simulink model "matlab_simulation"  (R2015b)
settings: Solver=VariableStepAuto  StartTime=0  StopTime=0.8  FixedStep=0.001  RelTol=1e-3
libraries: fl_lib x14, nesl_utility x8, elec_lib x5
settings Model: Creator=User  LastModifiedBy=User

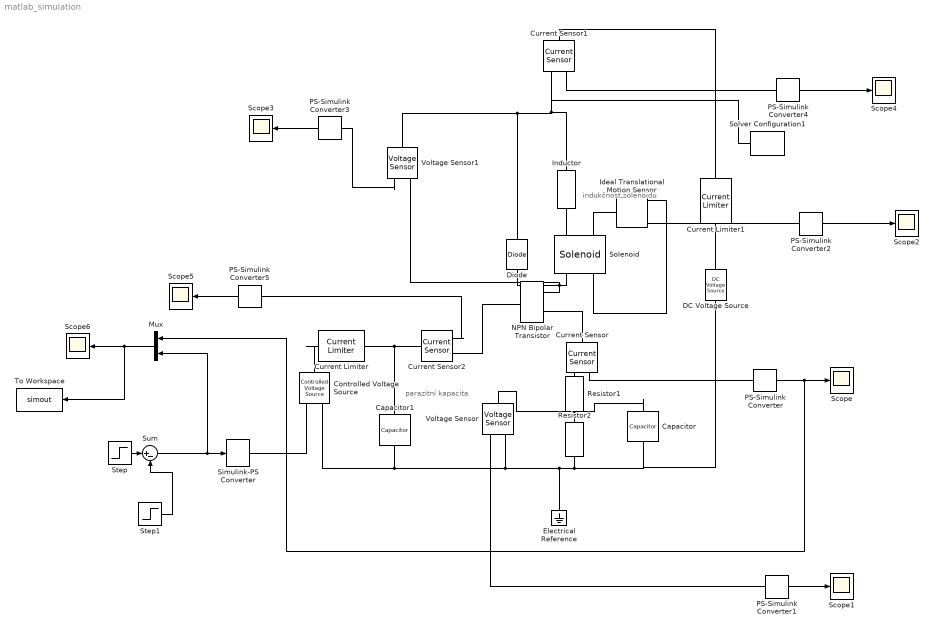
== system matlab_simulation ==
  note: parazitní kapacita
  note: indukčnost solenoidu
  Capacitor : fl_lib/Electrical/Electrical Elements/Capacitor  c=3.3e-3 F  r=1e-6 Ohm  g=0 1/Ohm  i_specify=off  i_priority=None  i=0 A  v_specify=off  v_priority=None  v=0 V  vc_specify=off  vc_priority=None  vc=0 V
  Capacitor1 : fl_lib/Electrical/Electrical Elements/Capacitor  c=50e-9 F  r=1e-6 Ohm  g=0 1/Ohm  i_specify=off  i_priority=None  i=0 A  v_specify=off  v_priority=None  v=0 V  vc_specify=off  vc_priority=None  vc=0 V
  Controlled Voltage Source : fl_lib/Electrical/Electrical Sources/Controlled Voltage Source
  Current Limiter : elec_lib/Semiconductor Devices/Current Limiter  iLim=20 mA  vLim=0.1 V  gLim=1e-9 1/Ohm  thermal_mass=100 J/K  initial_temperature=298.15 K
  Current Limiter1 : elec_lib/Semiconductor Devices/Current Limiter  iLim=2 A  vLim=0.1 V  gLim=1e-9 1/Ohm  thermal_mass=100 J/K  initial_temperature=298.15 K
  Current Sensor : fl_lib/Electrical/Electrical Sensors/Current Sensor
  Current Sensor1 : fl_lib/Electrical/Electrical Sensors/Current Sensor
  Current Sensor2 : fl_lib/Electrical/Electrical Sensors/Current Sensor
  DC Voltage Source : fl_lib/Electrical/Electrical Sources/DC Voltage Source  v0=12 V
  Diode : elec_lib/Semiconductor Devices/Diode  ModelType=1  Vf=0.6 V  Ron=0.3 Ohm  Goff=1e-8 S  Rz=0.3 Ohm  Vz=50 V  C_PWL=50 pF  prmExp=1  I12=[ 0.0137 0.545 ] A  V12=[ 0.6 0.7 ] V  I1=0.0137 A  V1=0.6 V  RS=0.01 Ohm  IS=1e-12 A  Tmeas=25 C  ec=1  BV=Inf V  C_param=1  CJ0=5 pF  VJ=1 V  Mgrad=0.5  Vvec=[ 0.1 10 100 ] V  Cvec=[ 3.5 1 0.4 ] pF  FC=0.5  Q_param=1  Irrm=-7.15 A  iF=4 A  didt=-750 A/us  trr=115 ns  TT=50 ns  tau=100 ns  T_param=1  IS_T2=1.25e-7 A  I1_T2=0.245 A  V1_T2=0.5 V  Tmeas2=125 C  EG_param=1  EG=1.11 eV  XTI_param=1  XTI=3  dBVdT=0 V/K  Tdevice=25 C  Rth=[ 0 10 ] K/W  thermal_mass_parameterization=1  thermal_mass=[ 0 1 ] J/K  thermal_time_constant=[ 0 10 ] s  thermal_mass_initial_temperatures=[ 25 25 ] C
  Electrical Reference : fl_lib/Electrical/Electrical Elements/Electrical Reference
  Ideal Translational Motion Sensor : fl_lib/Mechanical/Mechanical Sensors/Ideal Translational Motion Sensor  offset=1 mm
  Inductor : fl_lib/Electrical/Electrical Elements/Inductor  l=2359.25 uH  r=0 Ohm  g=1e-9 1/Ohm  i_specify=off  i_priority=None  i=0 A  v_specify=off  v_priority=None  v=0 V  i_L_specify=off  i_L_priority=None  i_L=0 A
  Mux : Mux  Inputs=2
  NPN Bipolar Transistor : elec_lib/Semiconductor Devices/NPN Bipolar Transistor  parameterization=1  prmDatasheet=1  prmEquCoeff=1  BF=100  IS=1e-14 A  ec=1  VAF=200 V  hfe=88  hoe=5e-5 1/Ohm  Ic_h=150 mA  Vce_h=2 V  V1=1 V  I1=2 mA  BR=100  Tmeas=25 C  RC=0.01 Ohm  RE=1e-4 Ohm  RB=1 Ohm  C_BC=50 pF  C_BE=50 pF  TF=0 us  TR=0 us  hfe_T2=125  XTB=0  V1_T2=0.45 V  I1_T2=0.5 mA  Tmeas2=125 C  EG=1.11 eV  XTI=3  TdeviceDatasheet=25 C  TdeviceEquCoeff=25 C  Rth=[ 0 10 ] K/W  thermal_mass_parameterization=1  thermal_mass=[ 0 1 ] J/K  thermal_time_constant=[ 0 10 ] s  thermal_mass_initial_temperatures=[ 25 25 ] C
  PS-Simulink Converter{,1..5} (6 alike) : nesl_utility/PS-Simulink Converter  PhysicalDomain=network_engine_domain  SubClassName=ps_output  LeftPortType=input  RightPortType=output  PseudoPeriodic=off  Frequencies=[]  Unit=1  AffineConversion=off
  Resistor1 : fl_lib/Electrical/Electrical Elements/Resistor  R=3.3 Ohm  i_specify=off  i_priority=None  i=0 A  v_specify=off  v_priority=None  v=0 V
  Resistor2 : fl_lib/Electrical/Electrical Elements/Resistor  R=24 Ohm  i_specify=off  i_priority=None  i=0 A  v_specify=off  v_priority=None  v=0 V
  Scope{,1..6} (7 alike) : Scope
  Simulink-PS Converter : nesl_utility/Simulink-PS Converter  PhysicalDomain=network_engine_domain  SubClassName=ps_input  LeftPortType=input  RightPortType=output  PseudoPeriodic=off  Frequencies=[]  NoiseDistribution=none  NoiseParameters=[]  Unit=1  AffineConversion=off  InputFiltering=off  SimscapeFilterOrder=1  InputFilterTimeConstant=0.001  UdotUserProvided=1
  Solenoid : elec_lib/Actuators & Drivers/Translational Actuators/Solenoid  F12=[ 7.5 0.75 ] N  X12=[ 1 4 ] mm  K=200 N/m  Xzero=5 mm  lam=1 N/(m/s)  Mass=0.05 kg  Vdc=5 V  Imax=1.1 A  Xmax=Inf mm  X0=5 mm  K_endstop=1e+6 N/m  D_endstop=500 N/(m/s)  alpha=0.00393 1/K  Tmeas=25 C  thermal_mass=100 J/K  initial_temperature=25 C
  Solver Configuration1 : nesl_utility/Solver Configuration  PhysicalDomain=network_engine_domain  SubClassName=solver  LeftPortType=input  RightPortType=generic  Accelerate=off  Tones=[]  Harmonics=[]  SimulateNoise=off  Profile=off  UseLocalSampling=off  EnableSwitchedLinearOptims=on  FrequencyDomain=off  UseCCode=off  RelTol=0.001  AbsTol=1e-06  MinStep=1e-09  ToWorkspace=off  RevertToSquareIcSolve=off  NumHomotopyIterations=100  PhasorMode=off  PhasorModeNumHarmonics=1  DoDC=off  ResidualTolerance=1e-09  UseLocalSolver=off  LocalSolverChoice=NE_BACKWARD_EULER_ADVANCER  LocalSolverSampleTime=0.001  DoFixedCost=off  MaxNonlinIter=3  MaxModeIter=2  LinearAlgebra=Sparse  DelaysMemoryBudget=1024  AutomaticFiltering=on  FilteringTimeConstant=0.001
  Step : Step  Time=0.52  After=5  SampleTime=0
  Step1 : Step  Time=0.6  After=5  SampleTime=0
  Sum : Sum  Inputs=|+-
  To Workspace : ToWorkspace  VariableName=simout  SaveFormat=Structure With Time  SampleTime=-1
  Voltage Sensor : fl_lib/Electrical/Electrical Sensors/Voltage Sensor
  Voltage Sensor1 : fl_lib/Electrical/Electrical Sensors/Voltage Sensor
  wires:
  PS-Simulink Converter1/1 -> Scope1/1
  PS-Simulink Converter3/1 -> Scope3/1
  Step/1 -> Sum/1
  Sum/1 -> Mux/2, Simulink-PS Converter/1
  Step1/1 -> Sum/2
  PS-Simulink Converter4/1 -> Scope4/1
  PS-Simulink Converter5/1 -> Scope5/1
  PS-Simulink Converter2/1 -> Scope2/1
  Mux/1 -> To Workspace/1, Scope6/1
  PS-Simulink Converter/1 -> Mux/1, Scope/1
  connections:
  Electrical Reference/LConn1 -- DC Voltage Source/RConn1 -- Capacitor/RConn1 -- Resistor2/RConn1 -- Voltage Sensor/RConn2 -- Capacitor1/RConn1 -- Controlled Voltage Source/RConn2
  NPN Bipolar Transistor/RConn2 -- Current Sensor/LConn1
  NPN Bipolar Transistor/RConn1 -- Voltage Sensor1/RConn2 -- Diode/LConn1 -- Solenoid/RConn1
  Diode/RConn1 -- Voltage Sensor1/LConn1 -- Inductor/LConn1 -- Current Sensor1/RConn2 -- Solver Configuration1/RConn1
  PS-Simulink Converter/LConn1 -- Current Sensor/RConn1
  Controlled Voltage Source/RConn1 -- Simulink-PS Converter/RConn1
  PS-Simulink Converter1/LConn1 -- Voltage Sensor/RConn1
  Current Sensor/RConn2 -- Resistor1/LConn1
  PS-Simulink Converter2/LConn1 -- Ideal Translational Motion Sensor/RConn3
  Solenoid/LConn2 -- Ideal Translational Motion Sensor/LConn1
  Solenoid/RConn2 -- Ideal Translational Motion Sensor/RConn1
  Resistor2/LConn1 -- Capacitor/LConn1 -- Voltage Sensor/LConn1 -- Resistor1/RConn1
  Voltage Sensor1/RConn1 -- PS-Simulink Converter3/LConn1
  PS-Simulink Converter4/LConn1 -- Current Sensor1/RConn1
  Current Sensor2/RConn2 -- NPN Bipolar Transistor/LConn1
  Current Sensor2/RConn1 -- PS-Simulink Converter5/LConn1
  Current Limiter/LConn1 -- Controlled Voltage Source/LConn1
  Current Limiter1/LConn1 -- DC Voltage Source/LConn1
  Current Limiter1/RConn1 -- Current Sensor1/LConn1
  Inductor/RConn1 -- Solenoid/LConn1
  Current Limiter/RConn1 -- Current Sensor2/LConn1 -- Capacitor1/LConn1
